simulink model "Argus_Simulink"  (R2021a)
settings: Solver=FixedStepAuto  StartTime=0.0  StopTime=5  FixedStep=Ts  RelTol=1e-3
values from neighbouring files (symbols this model uses):
  cog_mean = [-5.26624811124 -5.58012140225 -5.91171930264 -6.24331720303 -6.56162164639 -6.78761041592 -6.82232110928 -6.72852838467 -6.60371759366 -6.49736993741 -6.41834772061 -6.3873296542 ... (16721 elements, 16721x1)]    [cogging_data.mat]
  cog_pos = cog_pos*1000    [Argus_Parameters.m]    (also in cogging_data.mat = [-0.209006786426 -0.208981911621 -0.208956994531 -0.20893205)
  cor_fac = 1    [Argus_Parameters.m]
  COUNTS_PER_MM = 2500*2^12    (= 10240000)    [Argus_Parameters.m]
  IKP = 600    [Argus_Parameters.m]
  Ka_ff = SLAFF/2e7    [scale_gains.m]
  Ki = param(3)    [costfun_ARGUS_sim.m]    (also in scale_gains.m = SLVKI/2^16)
  Kp = param(1)    [costfun_ARGUS_sim.m]    (also in scale_gains.m = SLPKP)
  Kv = param(2)    [costfun_ARGUS_sim.m]    (also in scale_gains.m = SLVKP*scal_fac*SLVRAT/(1024))
  Kv_ff = 1    [Argus_Parameters.m]
  MFLAGS14 = 1    [Argus_Parameters.m]
  MFLAGS15 = 0    [Argus_Parameters.m]
  MFLAGS16 = 1    [Argus_Parameters.m]
  MFLAGS26 = 0    [Argus_Parameters.m]
  pos_os = 8.5    [Argus_Parameters.m]
  RPOS = s_curve(stepsize,vmax,acc,jerk,Ctime)    [Argus_RunSimulation.m]
  scale_cog = 1*scal_fac*Km*Lm    (= 1.0743808e-05)    [Argus_Parameters.m]
  SLVB0DD = 0.2    [Argus_Parameters.m]
  SLVB0DF = 750    [Argus_Parameters.m]
  SLVB0ND = 0.1    [Argus_Parameters.m]
  SLVB0NF = 750    [Argus_Parameters.m]
  SLVB1DD = 0.2    [Argus_Parameters.m]
  SLVB1DF = 450    [Argus_Parameters.m]
  SLVB1ND = 0.2    [Argus_Parameters.m]
  SLVB1NF = 500    [Argus_Parameters.m]
  SLVNATT = 2    [Argus_Parameters.m]
  SLVNFRQ = 520    [Argus_Parameters.m]
  SLVNWID = 30    [Argus_Parameters.m]
  SLVSOF = 1000    [Argus_Parameters.m]
  SLVSOFD = 0.707    [Argus_Parameters.m]
  V_LI = SLVLI/100    (= 0.5)    [Argus_Parameters.m]
  V_SF = 1    [Argus_Parameters.m]
  XVEL = COUNTS_PER_MM*3000    (= 30720000000)    [Argus_Parameters.m]
undefined symbols (not defined in the file or in its folder): Ctime, Ts
libraries: simulink x6, cstblocks x1
settings Model: Creator=CK  LastModifiedBy=chkoenig
settings SolverCC: AlgebraicLoopSolver=TrustRegion
settings DataIOCC: ReturnWorkspaceOutputs=off
settings DebuggingCC: SFMachineParentedDataDiag=warning  ArithmeticOperatorsInVariantConditions=warning
settings SFSimCC: SimUseLocalCustomCode=off  CustomCodeUndefinedFunction=UseInterfaceOnly
settings RTWCC: RTWUseLocalCustomCode=off

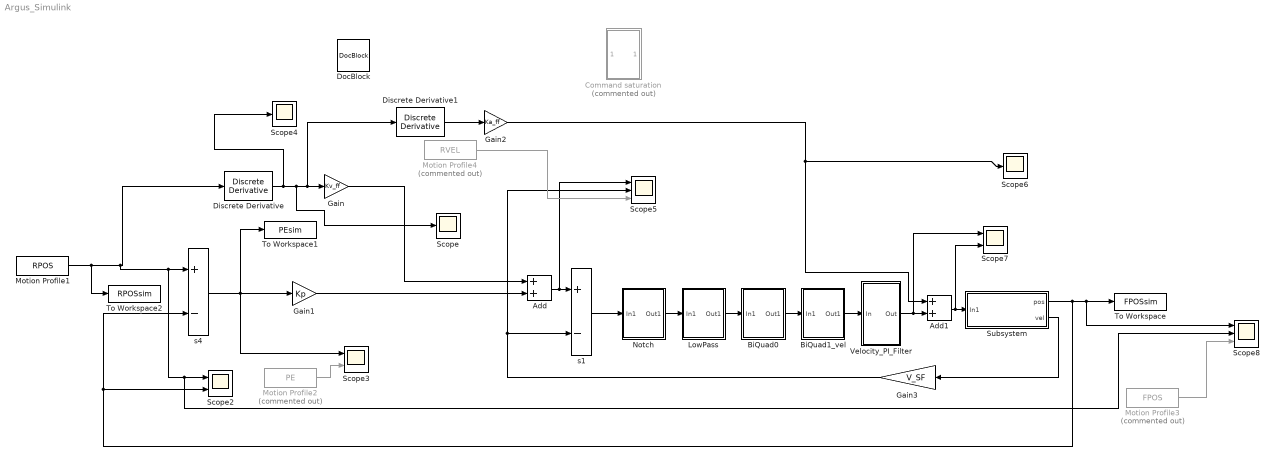
== system Argus_Simulink ==
  Add : Sum
  Add1 : Sum
  BiQuad0 : Subsystem
  BiQuad1_vel : Subsystem
  Command saturation : Subsystem  Commented=on
  Discrete Derivative : simulink/Discrete/Discrete Derivative  gainval=1.0  ICPrevScaledInput=0  OutMin=[]  OutMax=[]  OutDataType=fixdt(1, 16)  OutScaling=2^-10  DoSatur=off
  Discrete Derivative1 : simulink/Discrete/Discrete Derivative  gainval=1.0  ICPrevScaledInput=0.0  OutMin=[]  OutMax=[]  OutDataType=fixdt(1, 16)  OutScaling=2^-10  DoSatur=off
  DocBlock : simulink/Model-Wide Utilities/DocBlock  DocumentType=Text
      content=|
      | Acceleration feedforward not tested and varyfied!!!
  Gain : Gain  Gain=Kv_ff
  Gain1 : Gain  Gain=Kp
  Gain2 : Gain  Gain=Ka_ff
  Gain3 : Gain  Gain=V_SF
  LowPass : Subsystem
  Motion Profile1 : FromWorkspace  VariableName=RPOS  OutDataTypeStr=double  OutputAfterFinalValue=Holding final value
  Motion Profile2 : FromWorkspace  Commented=on  VariableName=PE  Interpolate=off  OutputAfterFinalValue=Holding final value
  Motion Profile3 : FromWorkspace  Commented=on  VariableName=FPOS  Interpolate=off  OutputAfterFinalValue=Holding final value
  Motion Profile4 : FromWorkspace  Commented=on  VariableName=RVEL  SampleTime=Ctime  OutputAfterFinalValue=Holding final value
  Notch : Subsystem
  Scope : Scope
  Scope2 : Scope  NumInputPorts=2
  Scope3 : Scope  NumInputPorts=2
  Scope4 : Scope
  Scope5 : Scope  NumInputPorts=3
  Scope6 : Scope
  Scope7 : Scope  NumInputPorts=2
  Scope8 : Scope  NumInputPorts=3
  Subsystem : Subsystem
  To Workspace : ToWorkspace  VariableName=FPOSsim  SaveFormat=Structure With Time  SampleTime=-1
  To Workspace1 : ToWorkspace  VariableName=PEsim  SaveFormat=Structure With Time  SampleTime=-1
  To Workspace2 : ToWorkspace  VariableName=RPOSsim  SaveFormat=Structure With Time  SampleTime=-1
  Velocity_PI_Filter : Subsystem
  s1 : Sum  Inputs=+-  InputSameDT=on  SaturateOnIntegerOverflow=on  OutDataTypeStr=Inherit: Same as first input
  s4 : Sum  Inputs=+-  InputSameDT=on  SaturateOnIntegerOverflow=on  OutDataTypeStr=Inherit: Same as first input
  wires:
  Gain1/1 -> Add/2
  Add/1 -> Scope5/1, s1/1
  Notch/1(Out1) -> LowPass/1(In1)
  LowPass/1(Out1) -> BiQuad0/1(In1)
  BiQuad0/1(Out1) -> BiQuad1_vel/1(In1)
  Discrete Derivative1/1 -> Gain2/1
  BiQuad1_vel/1(Out1) -> Velocity_PI_Filter/1(In)
  Velocity_PI_Filter/1(Out) -> Scope7/1, Add1/2
  Add1/1 -> Scope7/2, Subsystem/1(In1)
  Subsystem/1(pos) -> s4/2, Scope2/2, Scope8/1, To Workspace/1
  s4/1 -> To Workspace1/1, Scope3/1, Gain1/1
  s1/1 -> Notch/1(In1)
  Subsystem/2(vel) -> Gain3/1
  Gain3/1 -> s1/2, Scope5/2
  Discrete Derivative/1 -> Scope4/1, Scope/1, Discrete Derivative1/1, Gain/1
  Motion Profile2/1 -> Scope3/2
  Motion Profile3/1 -> Scope8/3
  Motion Profile4/1 -> Scope5/3
  Gain/1 -> Add/1
  Gain2/1 -> Scope6/1, Add1/1
  Motion Profile1/1 -> To Workspace2/1, Discrete Derivative/1, Scope8/2, Scope2/1, s4/1

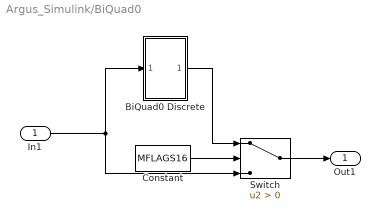
== system Argus_Simulink/BiQuad0 ==
  In1 : Inport
  BiQuad0 Discrete : Subsystem
  Constant : Constant  Value=MFLAGS16
  Switch : Switch  Criteria=u2 > Threshold
  Out1 : Outport  VectorParamsAs1DForOutWhenUnconnected=off
  wires:
  In1/1 -> Switch/3, BiQuad0 Discrete/1(In1)
  BiQuad0 Discrete/1(Out1) -> Switch/1
  Constant/1 -> Switch/2
  Switch/1 -> Out1/1

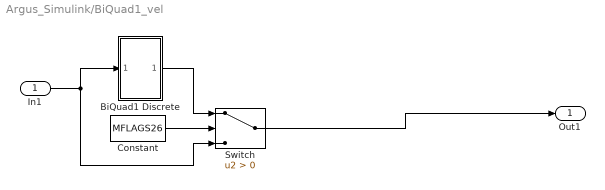
== system Argus_Simulink/BiQuad1_vel ==
  In1 : Inport
  BiQuad1 Discrete : Subsystem
  Constant : Constant  Value=MFLAGS26
  Switch : Switch  Criteria=u2 > Threshold
  Out1 : Outport  VectorParamsAs1DForOutWhenUnconnected=off
  wires:
  Switch/1 -> Out1/1
  BiQuad1 Discrete/1(Out1) -> Switch/1
  Constant/1 -> Switch/2
  In1/1 -> Switch/3, BiQuad1 Discrete/1(In1)

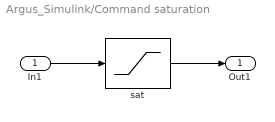
== system Argus_Simulink/Command saturation ==
  In1 : Inport
  "sat " : Saturate  UpperLimit=XVEL/COUNTS_PER_MM  LowerLimit=-XVEL/COUNTS_PER_MM
  Out1 : Outport  VectorParamsAs1DForOutWhenUnconnected=off
  wires:
  In1/1 -> "sat "/1
  "sat "/1 -> Out1/1

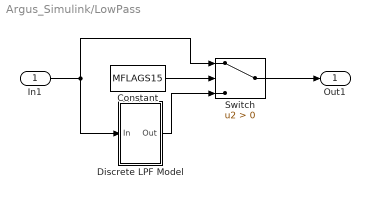
== system Argus_Simulink/LowPass ==
  In1 : Inport
  Constant : Constant  Value=MFLAGS15
  Discrete LPF Model : Subsystem
  Switch : Switch  Criteria=u2 > Threshold
  Out1 : Outport  VectorParamsAs1DForOutWhenUnconnected=off
  wires:
  Discrete LPF Model/1(Out) -> Switch/3
  In1/1 -> Switch/1, Discrete LPF Model/1(In)
  Constant/1 -> Switch/2
  Switch/1 -> Out1/1

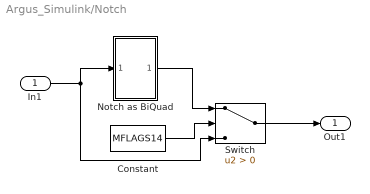
== system Argus_Simulink/Notch ==
  In1 : Inport
  Constant : Constant  Value=MFLAGS14
  Notch as BiQuad : Subsystem
  Switch : Switch  Criteria=u2 > Threshold
  Out1 : Outport  VectorParamsAs1DForOutWhenUnconnected=off
  wires:
  Notch as BiQuad/1(Out1) -> Switch/1
  In1/1 -> Notch as BiQuad/1(In1), Switch/3
  Constant/1 -> Switch/2
  Switch/1 -> Out1/1

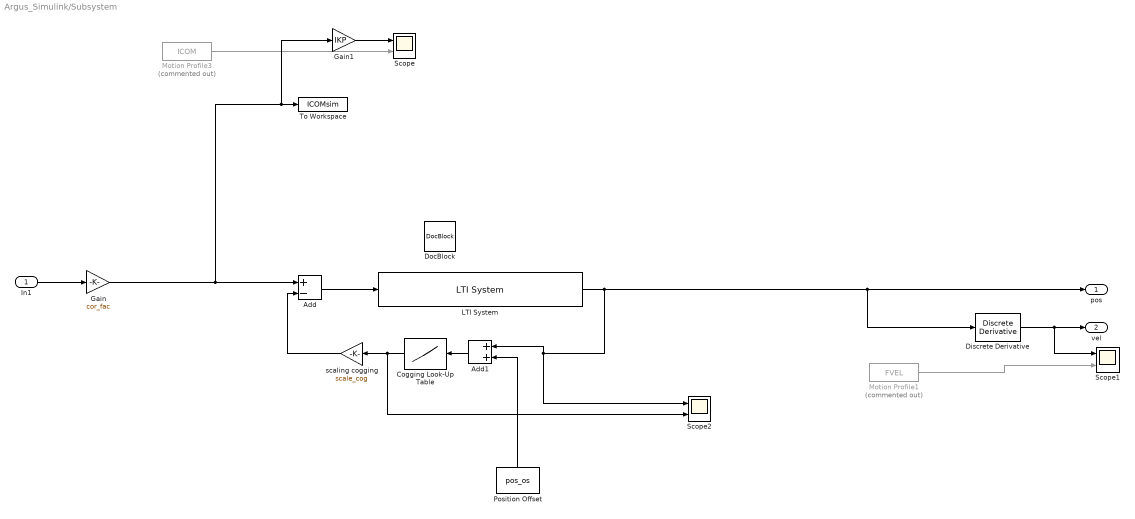
== system Argus_Simulink/Subsystem ==
  In1 : Inport
  Add : Sum  Inputs=+-
  Add1 : Sum
  Cogging Look-Up Table : Lookup  InputValues=cog_pos  Table=cog_mean  LookUpMeth=Interpolation-Use End Values  RndMeth=Nearest  SaturateOnIntegerOverflow=on
  Discrete Derivative : simulink/Discrete/Discrete Derivative  gainval=1.0  ICPrevScaledInput=RPOS(1,2)/Ts  OutMin=[]  OutMax=[]  OutDataType=fixdt(1, 16)  OutScaling=2^-10  DoSatur=off
  DocBlock : simulink/Model-Wide Utilities/DocBlock  DocumentType=Text
      content=|
      | Deadtime not included!!!
  Gain : Gain  Gain=cor_fac
  Gain1 : Gain  Gain=IKP
  LTI System : cstblocks/LTI System  sys=sys_plant  IC=[]
  Motion Profile1 : FromWorkspace  Commented=on  VariableName=FVEL  Interpolate=off  OutputAfterFinalValue=Holding final value
  Motion Profile3 : FromWorkspace  Commented=on  VariableName=ICOM  Interpolate=off  OutputAfterFinalValue=Holding final value
  Position Offset : Constant  Value=pos_os
  Scope : Scope  NumInputPorts=2
  Scope1 : Scope  NumInputPorts=2
  Scope2 : Scope  NumInputPorts=2
  To Workspace : ToWorkspace  VariableName=ICOMsim  SaveFormat=Structure With Time  SampleTime=-1
  scaling cogging : Gain  Gain=scale_cog  SaturateOnIntegerOverflow=on  OutDataTypeStr=Inherit: Same as input  ParamDataTypeStr=Inherit: Same as input
  pos : Outport  VectorParamsAs1DForOutWhenUnconnected=off
  vel : Outport  Port=2  VectorParamsAs1DForOutWhenUnconnected=off
  wires:
  Discrete Derivative/1 -> Scope1/1, vel/1
  Motion Profile3/1 -> Scope/2
  In1/1 -> Gain/1
  Motion Profile1/1 -> Scope1/2
  Cogging Look-Up Table/1 -> Scope2/2, scaling cogging/1
  Add/1 -> LTI System/1
  Add1/1 -> Cogging Look-Up Table/1
  Position Offset/1 -> Add1/2
  scaling cogging/1 -> Add/2
  Gain1/1 -> Scope/1
  Gain/1 -> Add/1, Gain1/1, To Workspace/1
  LTI System/1 -> Discrete Derivative/1, pos/1, Add1/1, Scope2/1

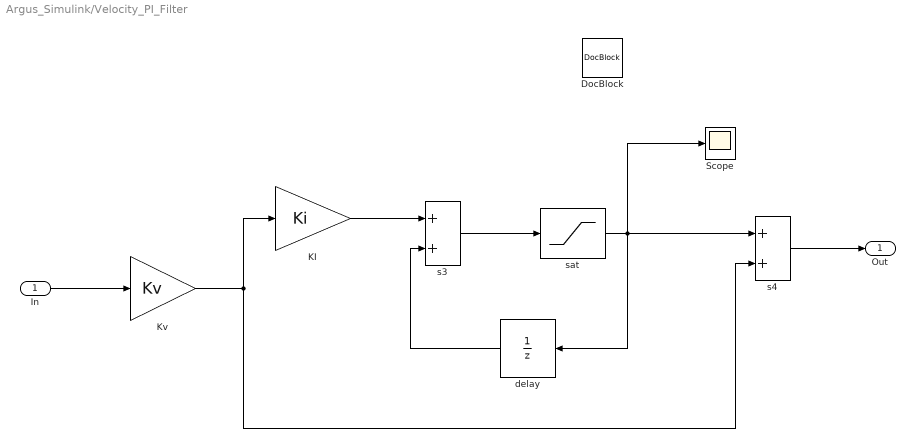
== system Argus_Simulink/Velocity_PI_Filter ==
  In : Inport
  DocBlock : simulink/Model-Wide Utilities/DocBlock  DocumentType=Text
      content=|
      | Saturation seems unrealistc!!!
  KI : Gain  Gain=Ki  SaturateOnIntegerOverflow=on  OutDataTypeStr=Inherit: Same as input  ParamDataTypeStr=Inherit: Same as input
  Kv : Gain  Gain=Kv  SaturateOnIntegerOverflow=on  OutDataTypeStr=Inherit: Same as input  ParamDataTypeStr=Inherit: Same as input
  Scope : Scope
  delay : UnitDelay  SampleTime=Ts  HasFrameUpgradeWarning=on
  s3 : Sum  InputSameDT=on  SaturateOnIntegerOverflow=on  OutDataTypeStr=Inherit: Same as first input
  s4 : Sum  InputSameDT=on  SaturateOnIntegerOverflow=on  OutDataTypeStr=Inherit: Same as first input
  "sat " : Saturate  UpperLimit=V_LI  LowerLimit=-V_LI
  Out : Outport  InitialOutput=0  VectorParamsAs1DForOutWhenUnconnected=off
  wires:
  In/1 -> Kv/1
  Kv/1 -> s4/2, KI/1
  s4/1 -> Out/1
  KI/1 -> s3/1
  s3/1 -> "sat "/1
  "sat "/1 -> s4/1, Scope/1, delay/1
  delay/1 -> s3/2

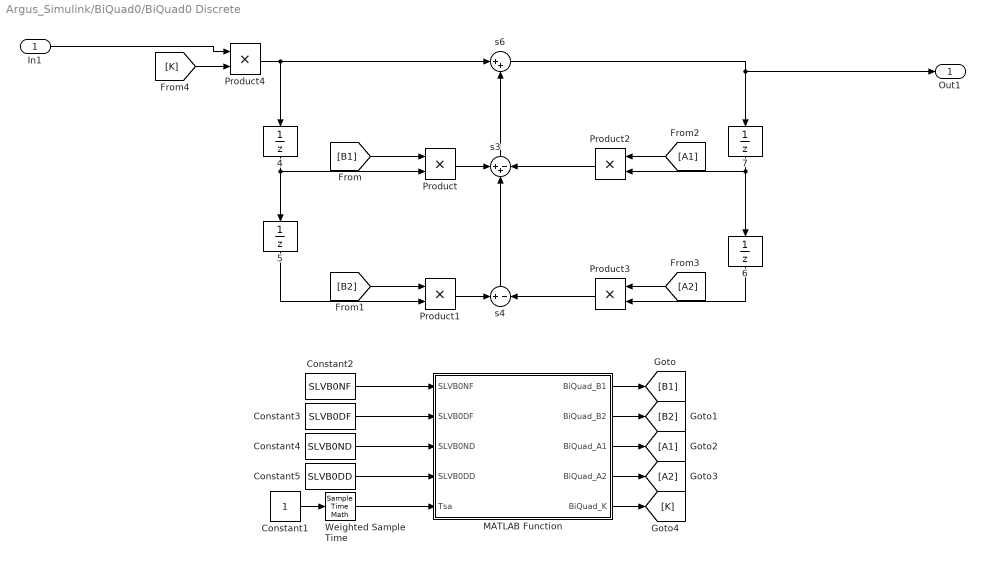
== system Argus_Simulink/BiQuad0/BiQuad0 Discrete ==
  In1 : Inport
   {4..7} (4 alike) : UnitDelay  SampleTime=Ts  HasFrameUpgradeWarning=on
  Constant1 : Constant
  Constant2 : Constant  Value=SLVB0NF
  Constant3 : Constant  Value=SLVB0DF
  Constant4 : Constant  Value=SLVB0ND
  Constant5 : Constant  Value=SLVB0DD
  MATLAB Function : MATLAB Function  TreatAsAtomicUnit=on
  Product{,1..4} (5 alike) : Product
  Weighted Sample Time : SampleTimeMath  TsampMathOp=Ts Only
  s3 : Sum  Inputs=++-  InputSameDT=on  SaturateOnIntegerOverflow=on  OutDataTypeStr=Inherit: Same as first input
  s4 : Sum  Inputs=+|-  InputSameDT=on  SaturateOnIntegerOverflow=on  OutDataTypeStr=Inherit: Same as first input
  s6 : Sum  Inputs=|++  InputSameDT=on  SaturateOnIntegerOverflow=on  OutDataTypeStr=Inherit: Same as first input
  Out1 : Outport  VectorParamsAs1DForOutWhenUnconnected=off
  wires:
  s4/1 -> s3/2
  " 6"/1 -> Product3/2
  " 4"/1 -> Product/2, " 5"/1
  s6/1 -> " 7"/1, Out1/1
  Constant4/1 -> MATLAB Function/3(SLVB0ND)
  MATLAB Function/4(BiQuad_A2) -> [A2]
  Weighted Sample Time/1 -> MATLAB Function/5(Tsa)
  Product/1 -> s3/1
  [B1] -> Product/1
  [B2] -> Product1/1
  [A1] -> Product2/1
  Product2/1 -> s3/3
  Product1/1 -> s4/1
  Constant1/1 -> Weighted Sample Time/1
  MATLAB Function/5(BiQuad_K) -> [K]
  Constant5/1 -> MATLAB Function/4(SLVB0DD)
  Constant2/1 -> MATLAB Function/1(SLVB0NF)
  MATLAB Function/2(BiQuad_B2) -> [B2]
  " 7"/1 -> Product2/2, " 6"/1
  s3/1 -> s6/2
  Constant3/1 -> MATLAB Function/2(SLVB0DF)
  " 5"/1 -> Product1/2
  MATLAB Function/3(BiQuad_A1) -> [A1]
  Product3/1 -> s4/2
  Product4/1 -> s6/1, " 4"/1
  In1/1 -> Product4/1
  [A2] -> Product3/1
  [K] -> Product4/2
  MATLAB Function/1(BiQuad_B1) -> [B1]

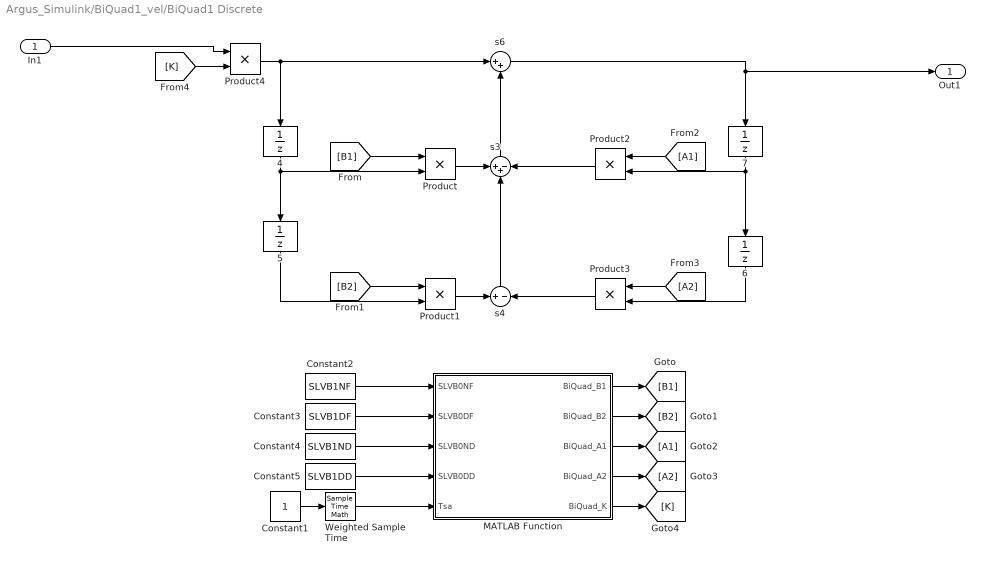
== system Argus_Simulink/BiQuad1_vel/BiQuad1 Discrete ==
  In1 : Inport
   {4..7} (4 alike) : UnitDelay  SampleTime=Ts  HasFrameUpgradeWarning=on
  Constant1 : Constant
  Constant2 : Constant  Value=SLVB1NF
  Constant3 : Constant  Value=SLVB1DF
  Constant4 : Constant  Value=SLVB1ND
  Constant5 : Constant  Value=SLVB1DD
  MATLAB Function : MATLAB Function  TreatAsAtomicUnit=on
  Product{,1..4} (5 alike) : Product
  Weighted Sample Time : SampleTimeMath  TsampMathOp=Ts Only
  s3 : Sum  Inputs=++-  InputSameDT=on  SaturateOnIntegerOverflow=on  OutDataTypeStr=Inherit: Same as first input
  s4 : Sum  Inputs=+|-  InputSameDT=on  SaturateOnIntegerOverflow=on  OutDataTypeStr=Inherit: Same as first input
  s6 : Sum  Inputs=|++  InputSameDT=on  SaturateOnIntegerOverflow=on  OutDataTypeStr=Inherit: Same as first input
  Out1 : Outport  VectorParamsAs1DForOutWhenUnconnected=off
  wires:
  s4/1 -> s3/2
  " 6"/1 -> Product3/2
  " 4"/1 -> Product/2, " 5"/1
  s6/1 -> " 7"/1, Out1/1
  Constant4/1 -> MATLAB Function/3(SLVB0ND)
  MATLAB Function/4(BiQuad_A2) -> [A2]
  Weighted Sample Time/1 -> MATLAB Function/5(Tsa)
  Product/1 -> s3/1
  [B1] -> Product/1
  [B2] -> Product1/1
  [A1] -> Product2/1
  Product2/1 -> s3/3
  Product1/1 -> s4/1
  Constant1/1 -> Weighted Sample Time/1
  MATLAB Function/5(BiQuad_K) -> [K]
  Constant5/1 -> MATLAB Function/4(SLVB0DD)
  Constant2/1 -> MATLAB Function/1(SLVB0NF)
  MATLAB Function/2(BiQuad_B2) -> [B2]
  " 7"/1 -> Product2/2, " 6"/1
  s3/1 -> s6/2
  Constant3/1 -> MATLAB Function/2(SLVB0DF)
  " 5"/1 -> Product1/2
  MATLAB Function/3(BiQuad_A1) -> [A1]
  Product3/1 -> s4/2
  Product4/1 -> s6/1, " 4"/1
  In1/1 -> Product4/1
  [A2] -> Product3/1
  [K] -> Product4/2
  MATLAB Function/1(BiQuad_B1) -> [B1]

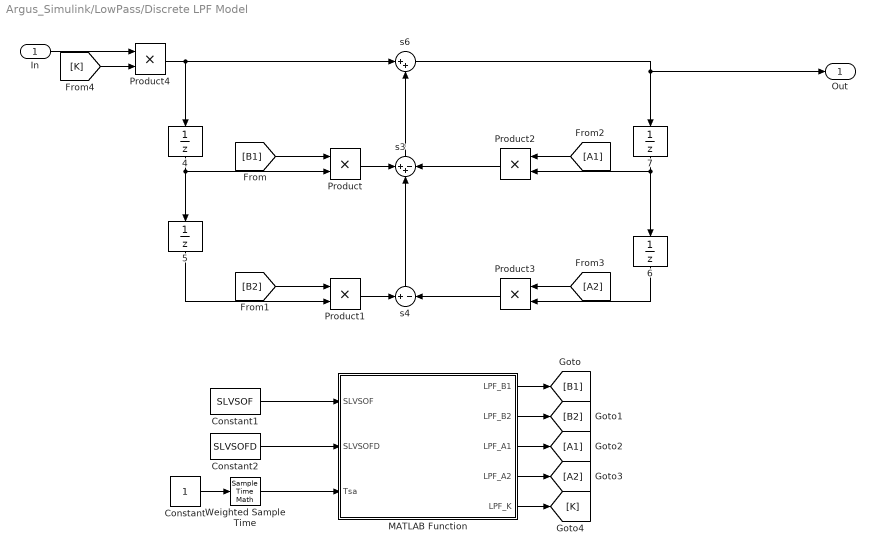
== system Argus_Simulink/LowPass/Discrete LPF Model ==
  In : Inport
   {4..7} (4 alike) : UnitDelay  SampleTime=Ts  HasFrameUpgradeWarning=on
  Constant : Constant
  Constant1 : Constant  Value=SLVSOF
  Constant2 : Constant  Value=SLVSOFD
  MATLAB Function : MATLAB Function  TreatAsAtomicUnit=on
  Product{,1..4} (5 alike) : Product
  Weighted Sample Time : SampleTimeMath  TsampMathOp=Ts Only
  s3 : Sum  Inputs=++-  InputSameDT=on  SaturateOnIntegerOverflow=on  OutDataTypeStr=Inherit: Same as first input
  s4 : Sum  Inputs=+|-  InputSameDT=on  SaturateOnIntegerOverflow=on  OutDataTypeStr=Inherit: Same as first input
  s6 : Sum  Inputs=|++  InputSameDT=on  SaturateOnIntegerOverflow=on  OutDataTypeStr=Inherit: Same as first input
  Out : Outport  InitialOutput=0  VectorParamsAs1DForOutWhenUnconnected=off
  wires:
  Product4/1 -> s6/1, " 4"/1
  In/1 -> Product4/1
  Product3/1 -> s4/2
  Product2/1 -> s3/3
  [K] -> Product4/2
  [A2] -> Product3/1
  [A1] -> Product2/1
  [B2] -> Product1/1
  [B1] -> Product/1
  Product/1 -> s3/1
  MATLAB Function/5(LPF_K) -> [K]
  Constant/1 -> Weighted Sample Time/1
  Weighted Sample Time/1 -> MATLAB Function/3(Tsa)
  Product1/1 -> s4/1
  " 6"/1 -> Product3/2
  s4/1 -> s3/2
  " 7"/1 -> Product2/2, " 6"/1
  " 5"/1 -> Product1/2
  " 4"/1 -> Product/2, " 5"/1
  s3/1 -> s6/2
  MATLAB Function/4(LPF_A2) -> [A2]
  s6/1 -> " 7"/1, Out/1
  MATLAB Function/3(LPF_A1) -> [A1]
  Constant1/1 -> MATLAB Function/1(SLVSOF)
  MATLAB Function/1(LPF_B1) -> [B1]
  MATLAB Function/2(LPF_B2) -> [B2]
  Constant2/1 -> MATLAB Function/2(SLVSOFD)

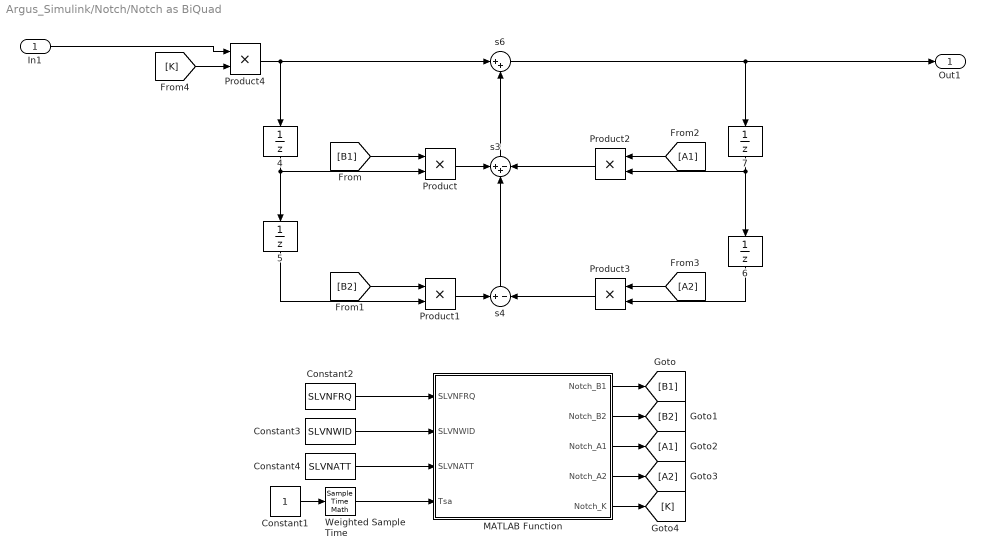
== system Argus_Simulink/Notch/Notch as BiQuad ==
  In1 : Inport
   {4..7} (4 alike) : UnitDelay  SampleTime=Ts  HasFrameUpgradeWarning=on
  Constant1 : Constant
  Constant2 : Constant  Value=SLVNFRQ
  Constant3 : Constant  Value=SLVNWID
  Constant4 : Constant  Value=SLVNATT
  MATLAB Function : MATLAB Function  TreatAsAtomicUnit=on
  Product{,1..4} (5 alike) : Product
  Weighted Sample Time : SampleTimeMath  TsampMathOp=Ts Only
  s3 : Sum  Inputs=++-  InputSameDT=on  SaturateOnIntegerOverflow=on  OutDataTypeStr=Inherit: Same as first input
  s4 : Sum  Inputs=+|-  InputSameDT=on  SaturateOnIntegerOverflow=on  OutDataTypeStr=Inherit: Same as first input
  s6 : Sum  Inputs=|++  InputSameDT=on  SaturateOnIntegerOverflow=on  OutDataTypeStr=Inherit: Same as first input
  Out1 : Outport  VectorParamsAs1DForOutWhenUnconnected=off
  wires:
  s4/1 -> s3/2
  " 6"/1 -> Product3/2
  " 4"/1 -> Product/2, " 5"/1
  s6/1 -> Out1/1, " 7"/1
  Constant4/1 -> MATLAB Function/3(SLVNATT)
  MATLAB Function/4(Notch_A2) -> [A2]
  Weighted Sample Time/1 -> MATLAB Function/4(Tsa)
  Product/1 -> s3/1
  [B1] -> Product/1
  [B2] -> Product1/1
  [A1] -> Product2/1
  Product2/1 -> s3/3
  Product1/1 -> s4/1
  Constant1/1 -> Weighted Sample Time/1
  MATLAB Function/5(Notch_K) -> [K]
  Constant2/1 -> MATLAB Function/1(SLVNFRQ)
  MATLAB Function/2(Notch_B2) -> [B2]
  " 7"/1 -> Product2/2, " 6"/1
  s3/1 -> s6/2
  Constant3/1 -> MATLAB Function/2(SLVNWID)
  " 5"/1 -> Product1/2
  MATLAB Function/3(Notch_A1) -> [A1]
  Product3/1 -> s4/2
  Product4/1 -> s6/1, " 4"/1
  In1/1 -> Product4/1
  [A2] -> Product3/1
  [K] -> Product4/2
  MATLAB Function/1(Notch_B1) -> [B1]

== matlab function Argus_Simulink/BiQuad0/BiQuad0 Discrete/MATLAB Function ==
  data: BiQuad_B1 output; BiQuad_B2 output; BiQuad_A1 output; SLVB0NF input; SLVB0DF input; SLVB0ND input; BiQuad_A2 output; SLVB0DD input; Tsa input; BiQuad_K output
function [BiQuad_B1, BiQuad_B2, BiQuad_A1, BiQuad_A2, BiQuad_K] = BiQuad_calc(SLVB0NF, SLVB0DF, SLVB0ND, SLVB0DD, Tsa)



wn = 2*pi*SLVB0NF;
wd = 2*pi*SLVB0DF;

zn = SLVB0ND;
zd = SLVB0DD;



if(zd<=1)
    BiQuad_A1 = -2*exp(-zd*wd*Tsa)*cos( wd*Tsa*sqrt(abs(1-zd^2)));
else
    BiQuad_A1 = -2*exp(-zd*wd*Tsa)*cosh(wd*Tsa*sqrt(abs(1-zd^2)));
end

BiQuad_A2 = exp(-2*zd*wd*Tsa);

if(zn<=1)
    BiQuad_B1 = -2*exp(-zn*wn*Tsa)*cos( wn*Tsa*sqrt(abs(1-zn^2)));
else
    BiQuad_B1 = -2*exp(-zn*wn*Tsa)*cosh(wn*Tsa*sqrt(abs(1-zn^2)));
end

BiQuad_B2 = exp(-2*zn*wn*Tsa);

BiQuad_K = (1+BiQuad_B1+BiQuad_B2)\(1+BiQuad_A1+BiQuad_A2);

== matlab function Argus_Simulink/BiQuad1_vel/BiQuad1 Discrete/MATLAB Function ==
  data: BiQuad_B1 output; BiQuad_B2 output; BiQuad_A1 output; SLVB0NF input; SLVB0DF input; SLVB0ND input; BiQuad_A2 output; SLVB0DD input; Tsa input; BiQuad_K output
function [BiQuad_B1, BiQuad_B2, BiQuad_A1, BiQuad_A2, BiQuad_K] = BiQuad_calc(SLVB0NF, SLVB0DF, SLVB0ND, SLVB0DD, Tsa)



wn = 2*pi*SLVB0NF;
wd = 2*pi*SLVB0DF;

zn = SLVB0ND;
zd = SLVB0DD;



if(zd<=1)
    BiQuad_A1 = -2*exp(-zd*wd*Tsa)*cos( wd*Tsa*sqrt(abs(1-zd^2)));
else
    BiQuad_A1 = -2*exp(-zd*wd*Tsa)*cosh(wd*Tsa*sqrt(abs(1-zd^2)));
end

BiQuad_A2 = exp(-2*zd*wd*Tsa);

if(zn<=1)
    BiQuad_B1 = -2*exp(-zn*wn*Tsa)*cos( wn*Tsa*sqrt(abs(1-zn^2)));
else
    BiQuad_B1 = -2*exp(-zn*wn*Tsa)*cosh(wn*Tsa*sqrt(abs(1-zn^2)));
end

BiQuad_B2 = exp(-2*zn*wn*Tsa);

BiQuad_K = (1+BiQuad_B1+BiQuad_B2)\(1+BiQuad_A1+BiQuad_A2);

== matlab function Argus_Simulink/LowPass/Discrete LPF Model/MATLAB Function ==
  data: LPF_B1 output; LPF_B2 output; LPF_A1 output; SLVSOF input; SLVSOFD input; LPF_A2 output; Tsa input; LPF_K output
function [LPF_B1, LPF_B2, LPF_A1, LPF_A2, LPF_K] = LPF_calc(SLVSOF, SLVSOFD, Tsa)


wd = 2*pi*SLVSOF;
zd = SLVSOFD;




LPF_B1 = 0;
LPF_B2 = 0;


LPF_A1 = -2*exp(-zd*wd*Tsa)*cos( wd*Tsa*sqrt(abs(1-zd^2)));
LPF_A2 = exp(-2*zd*wd*Tsa);

LPF_K = 1+LPF_A1+LPF_A2;

== matlab function Argus_Simulink/Notch/Notch as BiQuad/MATLAB Function ==
  data: Notch_B1 output; Notch_B2 output; Notch_A1 output; SLVNFRQ input; SLVNWID input; SLVNATT input; Notch_A2 output; Tsa input; Notch_K output
function [Notch_B1, Notch_B2, Notch_A1, Notch_A2, Notch_K] = Notch_calc(SLVNFRQ, SLVNWID, SLVNATT, Tsa)



SLVNWID = min(SLVNWID, 1/3*SLVNFRQ);
Q = max(3, SLVNFRQ/SLVNWID);

SLVB0NF = SLVNFRQ;
SLVB0DF = SLVNFRQ;
SLVB0ND = 1/Q/2;
SLVB0DD = SLVNATT/Q/2;

%%
wn = 2*pi*SLVB0NF;
wd = 2*pi*SLVB0DF;

zn = SLVB0ND;
zd = SLVB0DD;



if(zd<=1)
    Notch_A1 = -2*exp(-zd*wd*Tsa)*cos( wd*Tsa*sqrt(abs(1-zd^2)));
else
    Notch_A1 = -2*exp(-zd*wd*Tsa)*cosh(wd*Tsa*sqrt(abs(1-zd^2)));
end

Notch_A2 = exp(-2*zd*wd*Tsa);

if(zn<=1)
    Notch_B1 = -2*exp(-zn*wn*Tsa)*cos( wn*Tsa*sqrt(abs(1-zn^2)));
else
    Notch_B1 = -2*exp(-zn*wn*Tsa)*cosh(wn*Tsa*sqrt(abs(1-zn^2)));
end

Notch_B2 = exp(-2*zn*wn*Tsa);

Notch_K = (1+Notch_B1+Notch_B2)\(1+Notch_A1+Notch_A2);
